simulink model "BMS_detect"  (R2019b)
settings: Solver=ode23  StartTime=0.0  StopTime=30  FixedStep=1e-6  RelTol=0.001
model workspace (MAT data in the model file):
  socvcb = containers.Map
  socvcb.serialization.keys = {}
  socvcb.serialization.values = {}
  socvcb.serialization.uniformity = 0
  socvcb.serialization.keyType = 'double'
  socvcb.serialization.valueType = 'any'
values from neighbouring files (symbols this model uses):
  cell_prop = struct    [data_load.m]    (also in extend_model_ini.m = data_load('Cell_data.xlsx'))
libraries: fl_lib x28, nesl_utility x4, simulink x1, hwlogiciolib x1
settings Model: Creator=ZHOU Jinhan  LastModifiedBy=ZHOU Jinhan
settings SolverCC: ZeroCrossAlgorithm=Adaptive  AlgebraicLoopSolver=LineSearch

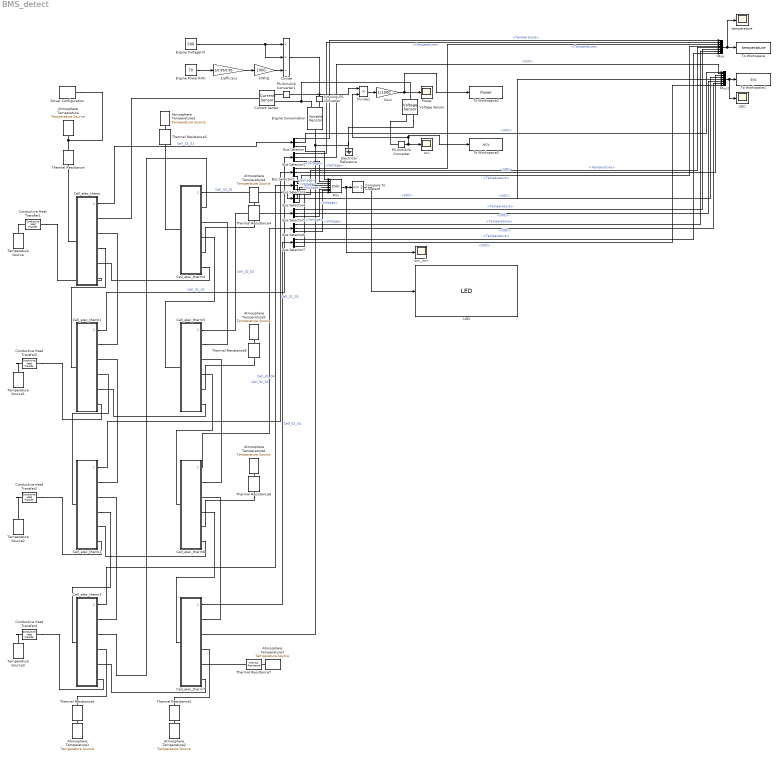
== system BMS_detect ==
  1/efficacy : Gain  Gain=1/0.95/0.95
  Atmosphere Temperature{,1..7} (8 alike) : fl_lib/Thermal/Thermal Sources/Temperature Source  temperature=cell_prop.T_ext K
      settings: SourceProductName=Simscape
  Bus Selector{,1..7} (8 alike) : BusSelector  OutputSignals=Temperature,SOC,Voltage
  Cell_elec_therm{,1..7} (8 alike) : Subsystem  ReferencedSubsystem=Cell_elec_therm
  Compare To Constant : simulink/Logic and Bit Operations/Compare To Constant  relop=<=  const=2  OutDataTypeStr=boolean
  Conductive Heat Transfer{1..2,4..5} (4 alike) : fl_lib/Thermal/Thermal Elements/Conductive Heat Transfer  area=0.1 m^2  thickness=0.1 m  th_cond=cell_prop.CFM*0.56657223796 W/(m*K)  T_specify=off  T_priority=None  T=0 K  T_nominal_specify=off  T_nominal_unit=K  T_nominal_value=1  Q_specify=off  Q_priority=None  Q=0 W  Q_nominal_specify=off  Q_nominal_unit=W  Q_nominal_value=1
      settings: SourceProductName=Simscape
  Current Sensor : fl_lib/Electrical/Electrical Sensors/Current Sensor
  Divide : Product  Inputs=**/
  Divide1 : Product  Inputs=**
  Electrical Reference : fl_lib/Electrical/Electrical Elements/Electrical Reference
  Engine Consomation : fl_lib/Electrical/Electrical Elements/Variable Resistor  Rmin=0 Ohm  i_specify=off  i_priority=None  i=0 A  i_nominal_specify=off  i_nominal_unit=A  i_nominal_value=1  v_specify=off  v_priority=None  v=0 V  v_nominal_specify=off  v_nominal_unit=V  v_nominal_value=1
  Engine Power(kW) : Constant  Value=70
  Engine Voltage(V) : Constant  Value=500
  Gain : Gain  Gain=1/1000
  LED : hwlogiciolib/LED  NumLeds=1  LastTargetBoard=None
      settings: SourceProductName=SoC Blockset  SourceProductBaseCode=HW
  Min : MinMax  Inputs=8
  Mux : Mux  Inputs=8
  Mux1 : Mux  Inputs=8
  PS-Simulink Converter : nesl_utility/PS-Simulink Converter  PhysicalDomain=network_engine_domain  SubClassName=ps_output  LeftPortType=input  RightPortType=output  PseudoPeriodic=off  Frequencies=[]  Unit=inherit  AffineConversion=off
  PS-Simulink Converter1 : nesl_utility/PS-Simulink Converter  PhysicalDomain=network_engine_domain  SubClassName=ps_output  LeftPortType=input  RightPortType=output  PseudoPeriodic=off  Frequencies=[]  Unit=inherit  AffineConversion=off
  Power : Scope
  SOC : Scope
  Simulink-PS Converter : nesl_utility/Simulink-PS Converter  PhysicalDomain=network_engine_domain  SubClassName=ps_input  LeftPortType=input  RightPortType=output  PseudoPeriodic=off  Frequencies=[]  NoiseDistribution=none  NoiseParameters=[]  Unit=1  AffineConversion=off  FilteringAndDerivatives=provide  SimscapeFilterOrder=1  InputFilterTimeConstant=0.001  UdotUserProvided=0
  Solver Configuration : nesl_utility/Solver Configuration  PhysicalDomain=network_engine_domain  SubClassName=solver  LeftPortType=input  RightPortType=generic  Tones=[]  Harmonics=[]  SimulateNoise=off  Profile=off  UseLocalSampling=off  EnableSwitchedLinearOptims=on  FrequencyDomain=off  UseCCode=off  RelTol=0.001  AbsTol=1e-06  MinStep=1e-09  ToWorkspace=off  RevertToSquareIcSolve=off  NumHomotopyIterations=100  PhasorMode=off  PhasorModeNumHarmonics=1  DoDC=off  ResidualTolerance=1e-06  UseLocalSolver=on  LocalSolverChoice=NE_BACKWARD_EULER_ADVANCER  LocalSolverSampleTime=0.001  DoFixedCost=off  MaxNonlinIter=3  MaxModeIter=2  LinearAlgebra=auto  EquationFormulation=NE_TIME_EF  DelaysMemoryBudget=1024  AutomaticFiltering=on  FilteringTimeConstant=0.001  PartitionStorageMethod=AS_NEEDED  PartitionMemoryBudget=1024  PartitionMethod=ROBUST
  Temperature Source{,1..3} (4 alike) : fl_lib/Thermal/Thermal Sources/Temperature Source  temperature=cell_prop.T_ext K
      settings: SourceProductName=Simscape
  Thermal Resistance{,1..7} (8 alike) : fl_lib/Thermal/Thermal Elements/Thermal Resistance  resistance=1/(1.006*1.202*0.028*50.4/60*1000) K/W  T_specify=off  T_priority=None  T=0 K  T_nominal_specify=off  T_nominal_unit=K  T_nominal_value=1  Q_specify=off  Q_priority=None  Q=0 W  Q_nominal_specify=off  Q_nominal_unit=W  Q_nominal_value=1
      settings: SourceProductName=Simscape  SourceProductBaseCode=SS
  To Workspace : ToWorkspace  VariableName=temperature  SaveFormat=Timeseries  SampleTime=-1
  To Workspace1 : ToWorkspace  VariableName=soc  SaveFormat=Timeseries  SampleTime=-1
  To Workspace2 : ToWorkspace  VariableName=Power  SaveFormat=Timeseries  SampleTime=-1
  To Workspace3 : ToWorkspace  VariableName=ocv  SaveFormat=Timeseries  SampleTime=-1
  Voltage Sensor : fl_lib/Electrical/Electrical Sensors/Voltage Sensor
  kWh2J : Gain  Gain=1000
  ocv : Scope
  ocv_min : Scope
  temperature : Scope
  wires:
  Cell_elec_therm/1 -> Bus Selector/1  "Cell_01_01"
  Cell_elec_therm1/1 -> Bus Selector1/1  "Cell_01_02"
  Cell_elec_therm3/1 -> Bus Selector3/1  "Cell_01_04"
  Cell_elec_therm2/1 -> Bus Selector2/1  "Cell_01_03"
  Cell_elec_therm4/1 -> Bus Selector4/1  "Cell_02_01"
  Cell_elec_therm5/1 -> Bus Selector5/1  "Cell_02_02"
  Cell_elec_therm6/1 -> Bus Selector6/1  "Cell_02_03"
  Cell_elec_therm7/1 -> Bus Selector7/1  "Cell_02_04"
  Engine Voltage(V)/1 -> Divide/1, Divide/2
  Engine Power(kW)/1 -> 1/efficacy/1
  Divide/1 -> Simulink-PS Converter/1
  kWh2J/1 -> Divide/3
  1/efficacy/1 -> kWh2J/1
  Compare To Constant/1 -> LED/1
  Min/1 -> ocv_min/1, Compare To Constant/1
  Bus Selector/2 -> Mux1/1  "<SOC>"
  Bus Selector/3 -> Min/1  "<Voltage>"
  Bus Selector1/3 -> Min/2  "<Voltage>"
  Bus Selector2/3 -> Min/3  "<Voltage>"
  Bus Selector3/3 -> Min/4  "<Voltage>"
  Bus Selector4/3 -> Min/5  "<Voltage>"
  Bus Selector5/3 -> Min/6  "<Voltage>"
  Bus Selector6/3 -> Min/7  "<Voltage>"
  Bus Selector7/3 -> Min/8  "<Voltage>"
  Bus Selector7/2 -> Mux1/8  "<SOC>"
  Bus Selector6/2 -> Mux1/7  "<SOC>"
  Bus Selector5/2 -> Mux1/6  "<SOC>"
  Bus Selector4/2 -> Mux1/5  "<SOC>"
  Bus Selector3/2 -> Mux1/4  "<SOC>"
  Bus Selector2/2 -> Mux1/3  "<SOC>"
  Bus Selector1/2 -> Mux1/2  "<SOC>"
  Mux/1 -> temperature/1, To Workspace/1
  Mux1/1 -> SOC/1, To Workspace1/1
  Bus Selector/1 -> Mux/1  "<Temperature>"
  Bus Selector1/1 -> Mux/2  "<Temperature>"
  Bus Selector2/1 -> Mux/3  "<Temperature>"
  Bus Selector3/1 -> Mux/4  "<Temperature>"
  Bus Selector4/1 -> Mux/5  "<Temperature>"
  Bus Selector5/1 -> Mux/6  "<Temperature>"
  Bus Selector6/1 -> Mux/7  "<Temperature>"
  Bus Selector7/1 -> Mux/8  "<Temperature>"
  PS-Simulink Converter1/1 -> Divide1/1
  PS-Simulink Converter/1 -> To Workspace3/1, Divide1/2, ocv/1
  Divide1/1 -> Gain/1
  Gain/1 -> To Workspace2/1, Power/1
  connections:
  Cell_elec_therm1/RConn1 -- Cell_elec_therm/RConn2
  Thermal Resistance/LConn1 -- Cell_elec_therm/LConn1
  Cell_elec_therm4/RConn5 -- Cell_elec_therm/RConn4
  Conductive Heat Transfer1/RConn1 -- Cell_elec_therm/RConn5
  Cell_elec_therm/RConn3 -- Cell_elec_therm1/LConn1
  Cell_elec_therm5/RConn5 -- Cell_elec_therm1/RConn4
  Cell_elec_therm2/RConn1 -- Cell_elec_therm1/RConn2
  Cell_elec_therm2/LConn1 -- Cell_elec_therm1/RConn3
  Conductive Heat Transfer5/RConn1 -- Cell_elec_therm1/RConn5
  Conductive Heat Transfer2/RConn1 -- Cell_elec_therm2/RConn5
  Cell_elec_therm3/RConn1 -- Cell_elec_therm2/RConn2
  Cell_elec_therm6/RConn5 -- Cell_elec_therm2/RConn4
  Thermal Resistance1/LConn1 -- Cell_elec_therm3/RConn3
  Cell_elec_therm3/RConn2 -- Cell_elec_therm4/RConn1
  Conductive Heat Transfer4/RConn1 -- Cell_elec_therm3/RConn5
  Cell_elec_therm2/RConn3 -- Cell_elec_therm3/LConn1
  Cell_elec_therm7/RConn5 -- Cell_elec_therm3/RConn4
  Cell_elec_therm6/LConn1 -- Cell_elec_therm5/RConn3
  Thermal Resistance4/LConn1 -- Cell_elec_therm4/RConn4
  Cell_elec_therm6/RConn1 -- Cell_elec_therm5/RConn2
  Thermal Resistance5/LConn1 -- Cell_elec_therm5/RConn4
  Engine Consomation/RConn1 -- Voltage Sensor/RConn2 -- Electrical Reference/LConn1 -- Cell_elec_therm7/RConn2
  Thermal Resistance6/LConn1 -- Cell_elec_therm6/RConn4
  Cell_elec_therm4/RConn3 -- Cell_elec_therm5/LConn1
  Cell_elec_therm5/RConn1 -- Cell_elec_therm4/RConn2
  Thermal Resistance7/LConn1 -- Cell_elec_therm7/RConn4
  Thermal Resistance2/LConn1 -- Cell_elec_therm7/RConn3
  Cell_elec_therm7/RConn1 -- Cell_elec_therm6/RConn2
  Cell_elec_therm6/RConn3 -- Cell_elec_therm7/LConn1
  Simulink-PS Converter/RConn1 -- Engine Consomation/LConn1
  Voltage Sensor/LConn1 -- Current Sensor/RConn2 -- Engine Consomation/LConn2
  Conductive Heat Transfer1/LConn1 -- Temperature Source/LConn1
  Conductive Heat Transfer5/LConn1 -- Temperature Source1/LConn1
  Conductive Heat Transfer2/LConn1 -- Temperature Source2/LConn1
  Conductive Heat Transfer4/LConn1 -- Temperature Source3/LConn1
  Atmosphere Temperature/LConn1 -- Solver Configuration/RConn1 -- Thermal Resistance/RConn1
  Atmosphere Temperature1/LConn1 -- Thermal Resistance1/RConn1
  Atmosphere Temperature2/LConn1 -- Thermal Resistance2/RConn1
  Atmosphere Temperature3/LConn1 -- Thermal Resistance3/RConn1
  Atmosphere Temperature4/LConn1 -- Thermal Resistance4/RConn1
  Atmosphere Temperature5/LConn1 -- Thermal Resistance5/RConn1
  Atmosphere Temperature6/LConn1 -- Thermal Resistance6/RConn1
  Atmosphere Temperature7/LConn1 -- Thermal Resistance7/RConn1
  Thermal Resistance3/LConn1 -- Cell_elec_therm4/LConn1
  PS-Simulink Converter/LConn1 -- Voltage Sensor/RConn1
  Current Sensor/LConn1 -- Cell_elec_therm/RConn1
  PS-Simulink Converter1/LConn1 -- Current Sensor/RConn1
